simulink subsystem "PX4_arm"  (R2024a)
settings: Solver=VariableStepAuto  StartTime=0.0  StopTime=10.0  RelTol=1e-3
libraries: px4uORBlib x1
settings Model: Creator=gurt1  LastModifiedBy=gurt1

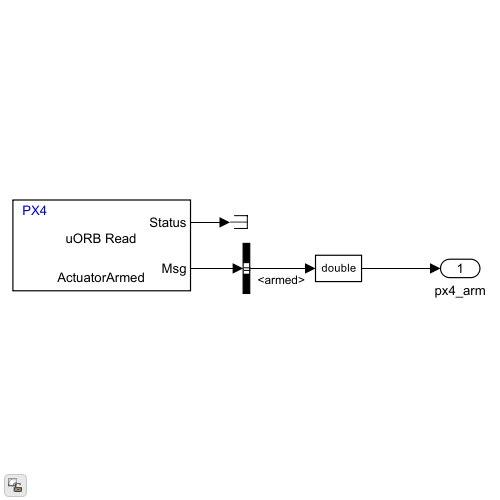
[thumbnail: Simulink's stored preview of the top-level diagram]
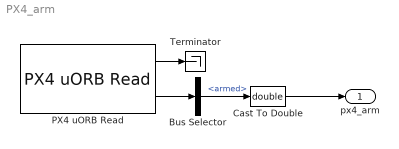
== system PX4_arm ==
  Bus Selector : BusSelector  OutputSignals=armed
  Cast To Double : DataTypeConversion  OutDataTypeStr=double  SaturateOnIntegerOverflow=off  RndMeth=Floor
  PX4 uORB Read : px4uORBlib/PX4 uORB Read  uORBTopic=ActuatorArmed  selectInstance=ActuatorArmed  SampleTime=-1  BlockingMode=off  BlockTimeout=1e-3
  Terminator : Terminator
  px4_arm : Outport
  wires:
  PX4 uORB Read/1 -> Terminator/1
  PX4 uORB Read/2 -> Bus Selector/1
  Bus Selector/1 -> Cast To Double/1  "<armed>"
  Cast To Double/1 -> px4_arm/1
